simulink model "sampled_polarity_integrator"  (R2017b)
settings: Solver=FixedStepAuto  StartTime=0.0  StopTime=10.0  FixedStep=0.01  RelTol=1e-3
settings Model: Creator=ernst  LastModifiedBy=ernst
settings DataIOCC: ExternalInput=[t__, u__]  LoadExternalInput=on  SaveFormat=StructureWithTime  SignalLogging=off  DSMLogging=off

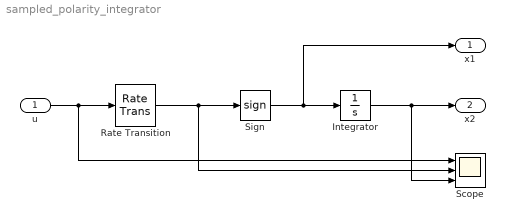
== system sampled_polarity_integrator ==
  u : Inport  Interpolate=off
  Integrator : Integrator
  Rate Transition : RateTransition  Integrity=off  OutPortSampleTime=1
  Scope : Scope  NumInputPorts=3
  Sign : Signum
  x1 : Outport
  x2 : Outport  Port=2
  wires:
  u/1 -> Scope/1, Rate Transition/1
  Sign/1 -> x1/1, Integrator/1
  Integrator/1 -> x2/1, Scope/3
  Rate Transition/1 -> Scope/2, Sign/1
